simulink model "mppt"  (R2020a)
settings: Solver=ode15s  StartTime=0.0  StopTime=parameters.sim_duration  FixedStep=1e-8  MaxStep=1e-7  RelTol=1e-3
undefined symbols (not defined in the file or in its folder): Ion, Lithium, parameters, sigbuilder_block
libraries: powerlib x24, simulink x5, powerlib_meascontrol x2, electricdrivelib x1, dspswit3 x1, re_lib x1
settings Model: SimulationMode=accelerator  Creator=HP  LastModifiedBy=HP

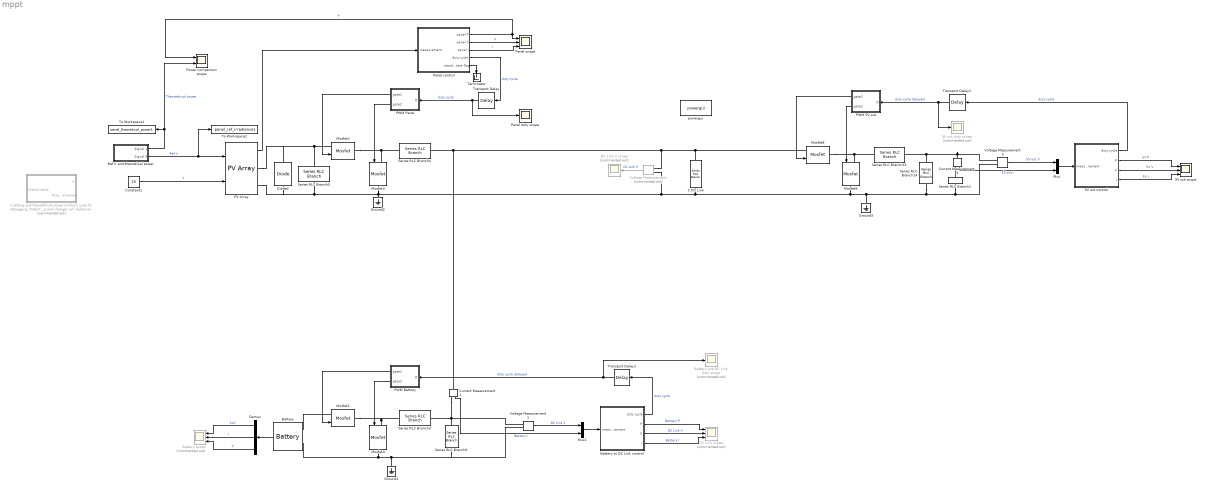
== system mppt ==
  5V out control : Subsystem
  5V out duty scope : Scope  Commented=on
  5V out scope : Scope  NumInputPorts=3
  Baterry scope : Scope  Commented=on  NumInputPorts=3
  Battery : electricdrivelib/Extra Sources/Battery  BatType=Lithium-Ion  ShowTempParam=off  ThermalPreset=no  ShowAgeParam=off  NomV=8  NomQ=2.6  SOC=50  Batt_Tr=30  PresetModel=off  MaxQ=2.6  MinV=6  FullV=9  Dis_rate=2.1304  R=0.019231  Normal_OP=2.3513  expZone="[8.5   2.12774]"  current=[6.5 13 32.5]  Units=Time  Tci=20  NomT=20  T2=-30  MaxQ2=4.8  FullV2=7.1  Normal_OP2=5.655  expZone2="[6.58           1]"  Rca=0.6  ti=2000  Dp=0  Neq0=0  Tsim=1e6  Ta1=25  Qeol=5.4*0.9  Reol=0.013333*1.2  Char_age=[2.3478, 3]  Dis_age=[2.3478, 10]  N1=1500  N2=10500  N3=1000  N4=1400  Ta2=45  N5=950
  Battery and DC Link duty scope : Scope  Commented=on
  Battery to DC Link control : Subsystem
  C DC Link : powerlib/Elements/Series RLC Branch  LConnTagsString=__new0  RConnTagsString=__new0  BranchType=RC  Resistance=0.01  Inductance=1e-3  SetiL0=off  InitialCurrent=0  Capacitance=400e-6  Setx0=off  InitialVoltage=0  Measurements=None
  Constant1 : Constant  Value=25
  Current Measurement1 : powerlib/Measurements/Current Measurement  PhasorSimulation=off  OutputType=Complex  PSBequivalent=0
  Current Measurement3 : powerlib/Measurements/Current Measurement  PhasorSimulation=off  OutputType=Complex  PSBequivalent=0
  DC Link V scope : Scope  Commented=on
  DC Link scope : Scope  Commented=on  NumInputPorts=3
  Demux : Demux  Outputs=3
  Diode2 : powerlib/Power Electronics/Diode  Ron=0.3  Lon=0  Vf=0.6  IC=0  UseSnubber=0  Rs=500  Cs=250e-9  Measurements=off
  Ground1 : powerlib/Elements/Ground  LConnTagsString=a
  Ground2 : powerlib/Elements/Ground  LConnTagsString=a
  Ground3 : powerlib/Elements/Ground  LConnTagsString=a
  Ir setting and theorethical power (A block used for debugging. Detects steady state and changes ref iradiance) : Subsystem  Commented=on
  Mosfet{1,4,8..9} (4 alike) : powerlib/Power Electronics/Mosfet  Ron=0.008  Lon=0  Rd=0.01  Vfd=1  IC=0  Rs=inf  Cs=inf  Measurements=off
  Mosfet2 : powerlib/Power Electronics/Mosfet  Ron=0.0029  Lon=0  Rd=0.01  Vfd=1  IC=0  Rs=inf  Cs=inf  Measurements=off
  Mosfet3 : powerlib/Power Electronics/Mosfet  Ron=0.0029  Lon=0  Rd=0.01  Vfd=1  IC=0  Rs=inf  Cs=inf  Measurements=off
  Mux : Mux  Inputs=2
  Mux1 : Mux  Inputs=2
  PV Array : re_lib/Solar/PV Array  Npar=1  Nser=1  PlotType=array @ 25 deg.C & specified irradiances  S_vec=[1000 800 500 400]  Temp_C_vec=[ 25 ]  ModuleName=User-defined  PlotWhenSelected=off  Pm=29.92  Ncell=36  Voc=21.9  Isc=1.84  Vm=17.6  Im=1.70  beta_Voc_pc=-0.33  alpha_Isc_pc=0.05  beta_Voc=-0.07227  alpha_Isc=0.00092  IL=1.8452  I0=2.0527e-11  nI=0.94005  Rsh=353.0773  Rs=1.0051  RobustModel=off  RobustCellTemperature=25  BAL=on  Tc=1e-8  Tfilter=5e-5
  PWM 5V out : Subsystem
  PWM Battery : Subsystem
  PWM Panel : Subsystem
  Panel control : Subsystem
  Panel duty scope : Scope
  Panel scope : Scope  NumInputPorts=3
  Power comparison scope : Scope  NumInputPorts=2
  Ref Ir and theoretical power : Subsystem  Tag=STV Subsys  LoadFcn=sigbuilder_block('load');  StartFcn=sigbuilder_block('start');  StopFcn=sigbuilder_block('stop');  ClipboardFcn=sigbuilder_block('clipboard');  mask(Sigbuilder block){tuvar=[0:10]}
      mask help: Simulink:masks:SigbuilderBlock_MD
      mask init:
      | if ~strcmp(get_param(bdroot(gcbh),'SimulationStatus'),'stopped') tuvar = sigbuilder_block('maskInit'); end
      settings: CopyFcn=sigbuilder_block('copy');  DeleteFcn=sigbuilder_block('delete');  ModelCloseFcn=sigbuilder_block('modelClose');  PreSaveFcn=sigbuilder_block('preSave');  PauseFcn=sigbuilder_block('pause');  ContinueFcn=sigbuilder_block('continue');  NameChangeFcn=sigbuilder_block('namechange');  OpenFcn=sigbuilder_block('open',[5.4 30 1141.2 522.6 ]);  CloseFcn=sigbuilder_block('close');
      mask Display: plot(0, 0, 100, 100,[2, 2, 32, 32, 2], [68, 8, 8, 68, 68],[32, 2], [38, 38], [32, 19, 2],[53, 60, 44], [32, 17, 17, 2],[16, 16, 31, 31]);txt = getActiveGroup(gcbh);text(2, 100, txt,'verticalAlignment', 'top');
  Series RLC Branch1 : powerlib/Elements/Series RLC Branch  LConnTagsString=__new0  RConnTagsString=__new0  BranchType=R  Resistance=2  Inductance=0  SetiL0=off  InitialCurrent=0  Capacitance=0  Setx0=off  InitialVoltage=0  Measurements=None
  Series RLC Branch13 : powerlib/Elements/Series RLC Branch  LConnTagsString=__new0  RConnTagsString=__new0  BranchType=RL  Resistance=0.01  Inductance=4.7e-6  SetiL0=off  InitialCurrent=0  Capacitance=1e-6  Setx0=off  InitialVoltage=0  Measurements=None
  Series RLC Branch14 : powerlib/Elements/Series RLC Branch  LConnTagsString=__new0  RConnTagsString=__new0  BranchType=RC  Resistance=0.01  Inductance=1e-3  SetiL0=off  InitialCurrent=0  Capacitance=47e-6  Setx0=off  InitialVoltage=0  Measurements=None
  Series RLC Branch3 : powerlib/Elements/Series RLC Branch  LConnTagsString=__new0  RConnTagsString=__new0  BranchType=RL  Resistance=0.01  Inductance=4.7e-6  SetiL0=off  InitialCurrent=0  Capacitance=1e-6  Setx0=off  InitialVoltage=0  Measurements=None
  Series RLC Branch4 : powerlib/Elements/Series RLC Branch  LConnTagsString=__new0  RConnTagsString=__new0  BranchType=RL  Resistance=0.009  Inductance=11.3e-6  SetiL0=off  InitialCurrent=0  Capacitance=1e-6  Setx0=off  InitialVoltage=0  Measurements=None
  Series RLC Branch5 : powerlib/Elements/Series RLC Branch  LConnTagsString=__new0  RConnTagsString=__new0  BranchType=RC  Resistance=0.01  Inductance=1e-3  SetiL0=off  InitialCurrent=0  Capacitance=22e-6  Setx0=off  InitialVoltage=0  Measurements=None
  Series RLC Branch6 : powerlib/Elements/Series RLC Branch  LConnTagsString=__new0  RConnTagsString=__new0  BranchType=RC  Resistance=0.01  Inductance=1e-3  SetiL0=off  InitialCurrent=0  Capacitance=47e-6  Setx0=off  InitialVoltage=0  Measurements=None
  Terminator : Terminator
  To Workspace1 : ToWorkspace  VariableName=panel_theoretical_power1  SaveFormat=Timeseries  SampleTime=-1
  To Workspace2 : ToWorkspace  VariableName=panel_ref_irradiance1  SaveFormat=Timeseries  SampleTime=-1
  Transport Delay : TransportDelay  DelayTime=parameters.transport_delay
  Transport Delay1 : TransportDelay  DelayTime=parameters.transport_delay
  Transport Delay2 : TransportDelay  DelayTime=parameters.transport_delay
  Voltage Measurement : powerlib/Measurements/Voltage Measurement  Commented=on  PhasorSimulation=off  OutputType=Complex  PSBequivalent=0
  Voltage Measurement1 : powerlib/Measurements/Voltage Measurement  PhasorSimulation=off  OutputType=Complex  PSBequivalent=0
  Voltage Measurement3 : powerlib/Measurements/Voltage Measurement  PhasorSimulation=off  OutputType=Complex  PSBequivalent=0
  powergui : powerlib/powergui  Priority=1  SimulationMode=Continuous  SampleTime=1e-8  frequency=60  Iterations=50  frequencyindice=0  Pbase=100e6  ErrMax=1e-4  UnitsV=kV  UnitsW=MW  buscounter=0  FunctionMessages=off  echomessages=off  EnableUseOfTLC=off  CurrentSourceSwitches=off  DisableSnubberDevices=off  DisableRonSwitches=off  DisableVfSwitches=off  DisplayEquations=off  AutomaticDiscreteSolvers=off  SolverType=Tustin/Backward Euler (TBE)  Interpol=off  ExternalGateDelay=off  methode=off  Ts=100  x0status=blocks  SPID=on  SwTol=0  HookPort=off  NonlinearTolerance=1e-4  nMaxIteration=100  ContinueOnMaxIteration=off  RestoreLinks=warning  ResistiveCurrentMeasurement=off  Frange=[0:2:500]  Ylog=off  Xlog=on  ShowGrid=off  save=off  variable=ZData  structure=0  ZoomFFT=off  StartTime=0.0  cycles=1  DisplayStyle=1  fundamental=60  FreqAxis=off  MaxFrequency=1000  frequencyindicesteady=1  RmsSteady=1  display=off
  wires:
  Constant1/1 -> PV Array/2  "T"
  PWM Panel/1(gate1) -> Mosfet2/1
  PWM Panel/2("gate2 ") -> Mosfet3/1
  PWM 5V out/1(gate1) -> Mosfet8/1
  Transport Delay2/1 -> PWM 5V out/1(D), 5V out duty scope/1  "duty cycle delayed"
  PWM 5V out/2("gate2 ") -> Mosfet9/1
  Voltage Measurement/1 -> DC Link V scope/1  "DC Link V"
  Panel control/1(panel P) -> Power comparison scope/1, Panel scope/1  "P"
  Panel control/2(panel V) -> Panel scope/2  "V"
  Panel control/3(panel I) -> Panel scope/3  "I"
  Panel control/4(duty cycle) -> Transport Delay/1  "duty cycle"
  5V out control/1(duty cycle) -> Transport Delay2/1  "duty cycle"
  Voltage Measurement3/1 -> Mux/1  "5V out V"
  Current Measurement3/1 -> Mux/2  "5V out I"
  Mux/1 -> 5V out control/1(measurement)
  5V out control/2(P) -> 5V out scope/1  "5V P"
  5V out control/3(V) -> 5V out scope/2  "5V V"
  5V out control/4(I) -> 5V out scope/3  "5V I"
  Battery/1 -> Demux/1
  Demux/1 -> Baterry scope/1  "SoC"
  Demux/2 -> Baterry scope/2  "I"
  Demux/3 -> Baterry scope/3  "V"
  Battery to DC Link control/3(V) -> DC Link scope/2  "DC Link V"
  Battery to DC Link control/1(duty cycle) -> Transport Delay1/1  "duty cycle"
  Current Measurement1/1 -> Mux1/2  "Battery I"
  Voltage Measurement1/1 -> Mux1/1  "DC Link V"
  Mux1/1 -> Battery to DC Link control/1(measurement)
  Transport Delay1/1 -> PWM Battery/1(D), Battery and DC Link duty scope/1  "duty cycle delayed"
  PWM Battery/1(gate1) -> Mosfet1/1
  Battery to DC Link control/4(I) -> DC Link scope/3  "Battery I"
  Battery to DC Link control/2(P) -> DC Link scope/1  "Battery P"
  PWM Battery/2("gate2 ") -> Mosfet4/1
  Transport Delay/1 -> PWM Panel/1(D), Panel duty scope/1  "duty cycle"
  PV Array/1 -> Panel control/1(measurement)
  Ref Ir and theoretical power/1(Signal 1) -> To Workspace1/1, Power comparison scope/2  "Theorethical power"
  Panel control/5(steady state flag) -> Terminator/1
  Ref Ir and theoretical power/2(Signal 3) -> To Workspace2/1, PV Array/1  "Ref ir"
  connections:
  Mosfet2/LConn1 -- Diode2/RConn1 -- PV Array/RConn1 -- Series RLC Branch5/LConn1
  Mosfet2/RConn1 -- Series RLC Branch4/RConn1 -- Mosfet3/LConn1
  Voltage Measurement3/LConn2 -- Series RLC Branch1/RConn1 -- Series RLC Branch14/RConn1 -- Ground3/LConn1 -- Mosfet9/RConn1 -- Voltage Measurement/LConn2 -- Mosfet3/RConn1 -- Ground2/LConn1 -- Diode2/LConn1 -- PV Array/RConn2 -- Series RLC Branch5/RConn1 -- C DC Link/RConn1
  Mosfet8/RConn1 -- Series RLC Branch13/RConn1 -- Mosfet9/LConn1
  Voltage Measurement3/LConn1 -- Current Measurement3/LConn1 -- Series RLC Branch13/LConn1 -- Series RLC Branch14/LConn1
  Current Measurement3/RConn1 -- Series RLC Branch1/LConn1
  C DC Link/LConn1 -- Mosfet8/LConn1 -- Voltage Measurement/LConn1 -- Current Measurement1/LConn1 -- Series RLC Branch4/LConn1
  Mosfet4/LConn1 -- Series RLC Branch3/RConn1 -- Mosfet1/RConn1
  Mosfet1/LConn1 -- Battery/LConn1
  Mosfet4/RConn1 -- Voltage Measurement1/LConn2 -- Series RLC Branch6/RConn1 -- Ground1/LConn1 -- Battery/LConn2
  Voltage Measurement1/LConn1 -- Current Measurement1/RConn1 -- Series RLC Branch3/LConn1 -- Series RLC Branch6/LConn1

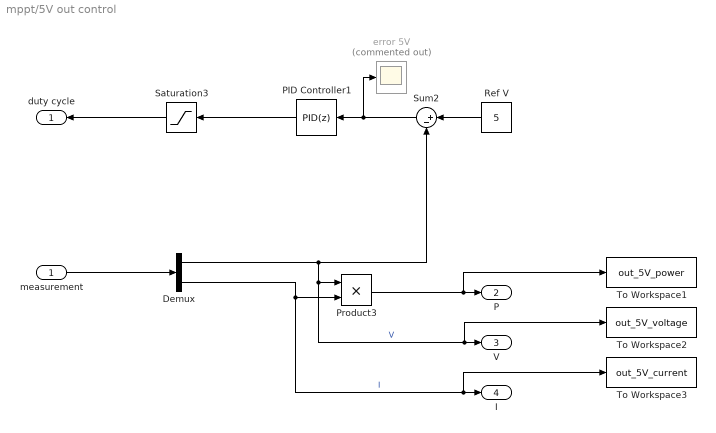
== system mppt/5V out control ==
  measurement : Inport
  Demux : Demux  Outputs=2
  PID Controller1 : simulink/Continuous/PID Controller  Controller=PID  Form=Parallel  TimeDomain=Discrete-time  UseExternalTs=off  SampleTime=parameters.sampling_time  IntegratorMethod=Forward Euler  FilterMethod=Forward Euler  ControllerParametersSource=internal  P=0.03  I=0.03*1e4  D=0  UseFilter=on  N=100  TunerSelectOption=Transfer Function Based (PID Tuner App)  InitialConditionSource=internal  InitialConditionForIntegrator=0  InitialConditionForFilter=0  DifferentiatorICPrevScaledInput=0  ExternalReset=none  TrackingMode=off  Kt=1  LimitOutput=off  UpperSaturationLimit=inf  LowerSaturationLimit=-inf  LinearizeAsGain=on  AntiWindupMode=none  Kb=1  POutMin=[]  POutMax=[]  IOutMin=[]  IOutMax=[]  DOutMin=[]  DOutMax=[]  NOutMin=[]  NOutMax=[]  SumOutMin=[]  SumOutMax=[]  SaturationOutMin=[]  SaturationOutMax=[]  PParamMin=[]  PParamMax=[]  IParamMin=[]  IParamMax=[]  DParamMin=[]  DParamMax=[]  NParamMin=[]  NParamMax=[]  KbParamMin=[]  KbParamMax=[]  KtParamMin=[]  KtParamMax=[]  KbOutMin=[]  KbOutMax=[]  KtOutMin=[]  KtOutMax=[]  IntegratorOutMin=[]  IntegratorOutMax=[]  FilterOutMin=[]  FilterOutMax=[]  SumI1OutMin=[]  SumI1OutMax=[]  SumI2OutMin=[]  SumI2OutMax=[]  SumI3OutMin=[]  SumI3OutMax=[]  SumI4OutMin=[]  SumI4OutMax=[]  SumDOutMin=[]  SumDOutMax=[]  DifferentiatorOutMin=[]  DifferentiatorOutMax=[]  FilterDiffOutCoefMin=[]  FilterDiffOutCoefMax=[]  ReciprocalOutMin=[]  ReciprocalOutMax=[]  SumDenOutMin=[]  SumDenOutMax=[]  SumNumOutMin=[]  SumNumOutMax=[]  DivideOutMin=[]  DivideOutMax=[]  UdiffTsProdOutMin=[]  UdiffTsProdOutMax=[]  NTsProdOutMin=[]  NTsProdOutMax=[]  UintegralTsProdOutMin=[]  UintegralTsProdOutMax=[]  UngainTsProdOutMin=[]  UngainTsProdOutMax=[]  IntegratorContinuousStateAttributes=''  IntegratorStateMustResolveToSignalObject=off  IntegratorRTWStateStorageClass=Auto  FilterContinuousStateAttributes=''  FilterStateMustResolveToSignalObject=off  FilterRTWStateStorageClass=Auto  ParallelPVariant=InternalParameters  IdealPVariant=Disabled  IVariant=InternalParameters  DVariant=InternalParameters  IntegratorVariant=Discrete  SatVariant=Disabled  AWVariant=Passthrough  PCopyVariant=Disabled  TRVariant=Disabled  FdbkBlocksVariant=Forward  IdealPFdbkVariant=Disabled  SatFdbkVariant=Disabled  DerivativeFilterVariant=ForwardEulerFilter  NVariant=InternalParameters  NCopyVariant=Disabled  FilterICVariant=InternalICsFilter  IntegratorICVariant=InternalICs  ExternalResetVariant=Disabled  TRSumVariant=Passthrough  SumFdbkVariant=Disabled  SumVariant=Sum_PID  TsampFilterVariant=InternalTs  TsampNgainVariant=Passthrough  TsampIntegralVariant=Passthrough
  Product3 : Product
  Ref V : Constant  Value=5
  Saturation3 : Saturate  UpperLimit=1  LowerLimit=0
  Sum2 : Sum  Inputs=|+-
  To Workspace1 : ToWorkspace  VariableName=out_5V_power  SaveFormat=Timeseries  SampleTime=-1
  To Workspace2 : ToWorkspace  VariableName=out_5V_voltage  SaveFormat=Timeseries  SampleTime=-1
  To Workspace3 : ToWorkspace  VariableName=out_5V_current  SaveFormat=Timeseries  SampleTime=-1
  error 5V : Scope  Commented=on
  duty cycle : Outport
  P : Outport  Port=2
  V : Outport  Port=3
  I : Outport  Port=4
  wires:
  Sum2/1 -> PID Controller1/1, error 5V/1
  PID Controller1/1 -> Saturation3/1
  Product3/1 -> To Workspace1/1, P/1
  Demux/1 -> Sum2/2, To Workspace2/1, V/1, Product3/1  "V"
  Ref V/1 -> Sum2/1
  Demux/2 -> To Workspace3/1, I/1, Product3/2  "I"
  Saturation3/1 -> duty cycle/1
  measurement/1 -> Demux/1

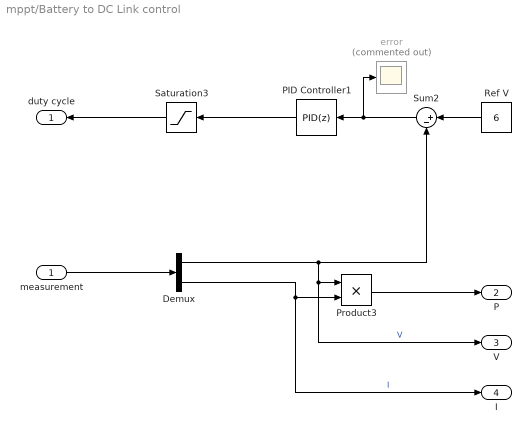
== system mppt/Battery to DC Link control ==
  measurement : Inport
  Demux : Demux  Outputs=2
  PID Controller1 : simulink/Continuous/PID Controller  Controller=PID  Form=Parallel  TimeDomain=Discrete-time  UseExternalTs=off  SampleTime=parameters.sampling_time  IntegratorMethod=Forward Euler  FilterMethod=Forward Euler  ControllerParametersSource=internal  P=0.03  I=0.03*1e4  D=0  UseFilter=on  N=100  TunerSelectOption=Transfer Function Based (PID Tuner App)  InitialConditionSource=internal  InitialConditionForIntegrator=0  InitialConditionForFilter=0  DifferentiatorICPrevScaledInput=0  ExternalReset=none  TrackingMode=off  Kt=1  LimitOutput=off  UpperSaturationLimit=inf  LowerSaturationLimit=-inf  LinearizeAsGain=on  AntiWindupMode=none  Kb=1  POutMin=[]  POutMax=[]  IOutMin=[]  IOutMax=[]  DOutMin=[]  DOutMax=[]  NOutMin=[]  NOutMax=[]  SumOutMin=[]  SumOutMax=[]  SaturationOutMin=[]  SaturationOutMax=[]  PParamMin=[]  PParamMax=[]  IParamMin=[]  IParamMax=[]  DParamMin=[]  DParamMax=[]  NParamMin=[]  NParamMax=[]  KbParamMin=[]  KbParamMax=[]  KtParamMin=[]  KtParamMax=[]  KbOutMin=[]  KbOutMax=[]  KtOutMin=[]  KtOutMax=[]  IntegratorOutMin=[]  IntegratorOutMax=[]  FilterOutMin=[]  FilterOutMax=[]  SumI1OutMin=[]  SumI1OutMax=[]  SumI2OutMin=[]  SumI2OutMax=[]  SumI3OutMin=[]  SumI3OutMax=[]  SumI4OutMin=[]  SumI4OutMax=[]  SumDOutMin=[]  SumDOutMax=[]  DifferentiatorOutMin=[]  DifferentiatorOutMax=[]  FilterDiffOutCoefMin=[]  FilterDiffOutCoefMax=[]  ReciprocalOutMin=[]  ReciprocalOutMax=[]  SumDenOutMin=[]  SumDenOutMax=[]  SumNumOutMin=[]  SumNumOutMax=[]  DivideOutMin=[]  DivideOutMax=[]  UdiffTsProdOutMin=[]  UdiffTsProdOutMax=[]  NTsProdOutMin=[]  NTsProdOutMax=[]  UintegralTsProdOutMin=[]  UintegralTsProdOutMax=[]  UngainTsProdOutMin=[]  UngainTsProdOutMax=[]  IntegratorContinuousStateAttributes=''  IntegratorStateMustResolveToSignalObject=off  IntegratorRTWStateStorageClass=Auto  FilterContinuousStateAttributes=''  FilterStateMustResolveToSignalObject=off  FilterRTWStateStorageClass=Auto  ParallelPVariant=InternalParameters  IdealPVariant=Disabled  IVariant=InternalParameters  DVariant=InternalParameters  IntegratorVariant=Discrete  SatVariant=Disabled  AWVariant=Passthrough  PCopyVariant=Disabled  TRVariant=Disabled  FdbkBlocksVariant=Forward  IdealPFdbkVariant=Disabled  SatFdbkVariant=Disabled  DerivativeFilterVariant=ForwardEulerFilter  NVariant=InternalParameters  NCopyVariant=Disabled  FilterICVariant=InternalICsFilter  IntegratorICVariant=InternalICs  ExternalResetVariant=Disabled  TRSumVariant=Passthrough  SumFdbkVariant=Disabled  SumVariant=Sum_PID  TsampFilterVariant=InternalTs  TsampNgainVariant=Passthrough  TsampIntegralVariant=Passthrough
  Product3 : Product
  Ref V : Constant  Value=6
  Saturation3 : Saturate  UpperLimit=1  LowerLimit=0
  Sum2 : Sum  Inputs=|+-
  "error " : Scope  Commented=on
  duty cycle : Outport
  P : Outport  Port=2
  V : Outport  Port=3
  I : Outport  Port=4
  wires:
  Sum2/1 -> PID Controller1/1, "error "/1
  PID Controller1/1 -> Saturation3/1
  Product3/1 -> P/1
  Demux/1 -> Sum2/2, V/1, Product3/1  "V"
  Ref V/1 -> Sum2/1
  Demux/2 -> I/1, Product3/2  "I"
  Saturation3/1 -> duty cycle/1
  measurement/1 -> Demux/1

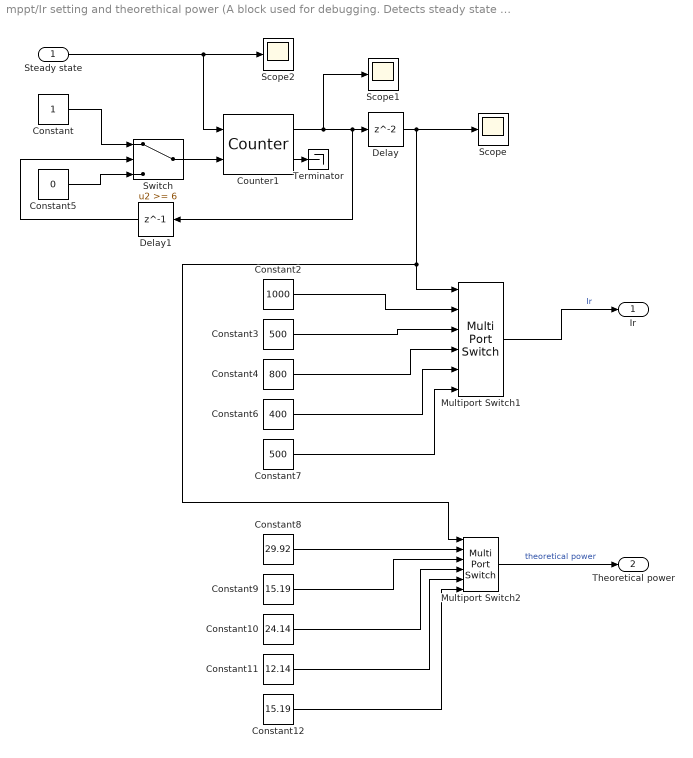
== system mppt/Ir setting and theorethical power (A block used for debugging. Detects steady state and changes ref iradiance) ==
  Steady state : Inport
  Constant : Constant
  Constant10 : Constant  Value=24.14
  Constant11 : Constant  Value=12.14
  Constant12 : Constant  Value=15.19
  Constant2 : Constant  Value=1000
  Constant3 : Constant  Value=500
  Constant4 : Constant  Value=800
  Constant5 : Constant  Value=0
  Constant6 : Constant  Value=400
  Constant7 : Constant  Value=500
  Constant8 : Constant  Value=29.92
  Constant9 : Constant  Value=15.19
  Counter1 : dspswit3/Counter  Direction=Up  CountEvent=Rising edge  CounterSize=User defined  MaxCount=255  InitialCount=1  Output=Count and Hit  HitValue=32  ResetInput=on  SamplesPerFrame=1  Ts=1  CntDtype=double  HitDtype=Logical
  Delay : Delay  InitialCondition=1
  Delay1 : Delay  DelayLength=1  InitialCondition=0
  Multiport Switch1 : MultiPortSwitch  Inputs=5
  Multiport Switch2 : MultiPortSwitch  Inputs=5
  Scope : Scope
  Scope1 : Scope
  Scope2 : Scope
  Switch : Switch  Threshold=6
  Terminator : Terminator
  Ir : Outport
  Theoretical power : Outport  Port=2
  wires:
  Constant9/1 -> Multiport Switch2/3
  Constant10/1 -> Multiport Switch2/4
  Delay/1 -> Multiport Switch1/1, Multiport Switch2/1, Scope/1
  Constant4/1 -> Multiport Switch1/4
  Constant11/1 -> Multiport Switch2/5
  Counter1/2 -> Terminator/1
  Constant/1 -> Switch/1
  Constant12/1 -> Multiport Switch2/6
  Counter1/1 -> Scope1/1, Delay1/1, Delay/1
  Constant8/1 -> Multiport Switch2/2
  Steady state/1 -> Scope2/1, Counter1/1
  Constant6/1 -> Multiport Switch1/5
  Constant5/1 -> Switch/3
  Constant7/1 -> Multiport Switch1/6
  Constant3/1 -> Multiport Switch1/3
  Constant2/1 -> Multiport Switch1/2
  Multiport Switch1/1 -> Ir/1  "Ir"
  Switch/1 -> Counter1/2
  Multiport Switch2/1 -> Theoretical power/1  "theoretical power"
  Delay1/1 -> Switch/2

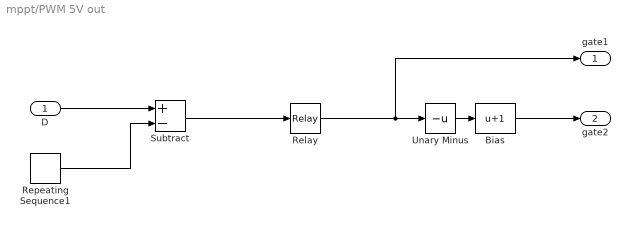
== system mppt/PWM 5V out ==
  D : Inport
  Bias : Bias  Bias=1
  Relay : Relay  OnSwitchValue=0  OffSwitchValue=0
  Repeating Sequence1 : simulink/Sources/Repeating Sequence  rep_seq_t=[0 1/300000]  rep_seq_y=[0 1]
  Subtract : Sum  Inputs=+-
  Unary Minus : UnaryMinus
  gate1 : Outport  VectorParamsAs1DForOutWhenUnconnected=off
  "gate2 " : Outport  Port=2  VectorParamsAs1DForOutWhenUnconnected=off
  wires:
  Relay/1 -> Unary Minus/1, gate1/1
  Subtract/1 -> Relay/1
  Unary Minus/1 -> Bias/1
  Bias/1 -> "gate2 "/1
  Repeating Sequence1/1 -> Subtract/2
  D/1 -> Subtract/1

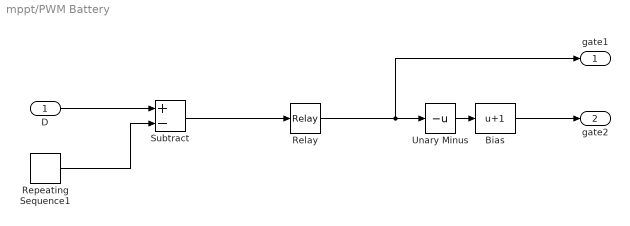
== system mppt/PWM Battery ==
  D : Inport
  Bias : Bias  Bias=1
  Relay : Relay  OnSwitchValue=0  OffSwitchValue=0
  Repeating Sequence1 : simulink/Sources/Repeating Sequence  rep_seq_t=[0 1/300000]  rep_seq_y=[0 1]
  Subtract : Sum  Inputs=+-
  Unary Minus : UnaryMinus
  gate1 : Outport  VectorParamsAs1DForOutWhenUnconnected=off
  "gate2 " : Outport  Port=2  VectorParamsAs1DForOutWhenUnconnected=off
  wires:
  Relay/1 -> Unary Minus/1, gate1/1
  Subtract/1 -> Relay/1
  Unary Minus/1 -> Bias/1
  Bias/1 -> "gate2 "/1
  Repeating Sequence1/1 -> Subtract/2
  D/1 -> Subtract/1

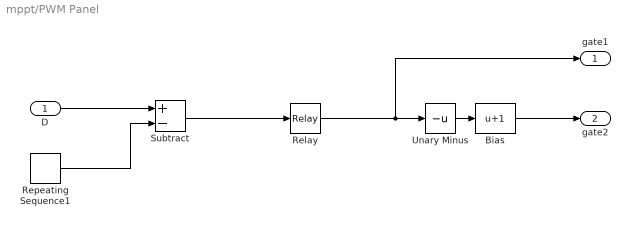
== system mppt/PWM Panel ==
  D : Inport
  Bias : Bias  Bias=1
  Relay : Relay  OnSwitchValue=0  OffSwitchValue=0
  Repeating Sequence1 : simulink/Sources/Repeating Sequence  rep_seq_t=[0 1/300000]  rep_seq_y=[0 1]
  Subtract : Sum  Inputs=+-
  Unary Minus : UnaryMinus
  gate1 : Outport  VectorParamsAs1DForOutWhenUnconnected=off
  "gate2 " : Outport  Port=2  VectorParamsAs1DForOutWhenUnconnected=off
  wires:
  Relay/1 -> Unary Minus/1, gate1/1
  Subtract/1 -> Relay/1
  Unary Minus/1 -> Bias/1
  Bias/1 -> "gate2 "/1
  Repeating Sequence1/1 -> Subtract/2
  D/1 -> Subtract/1

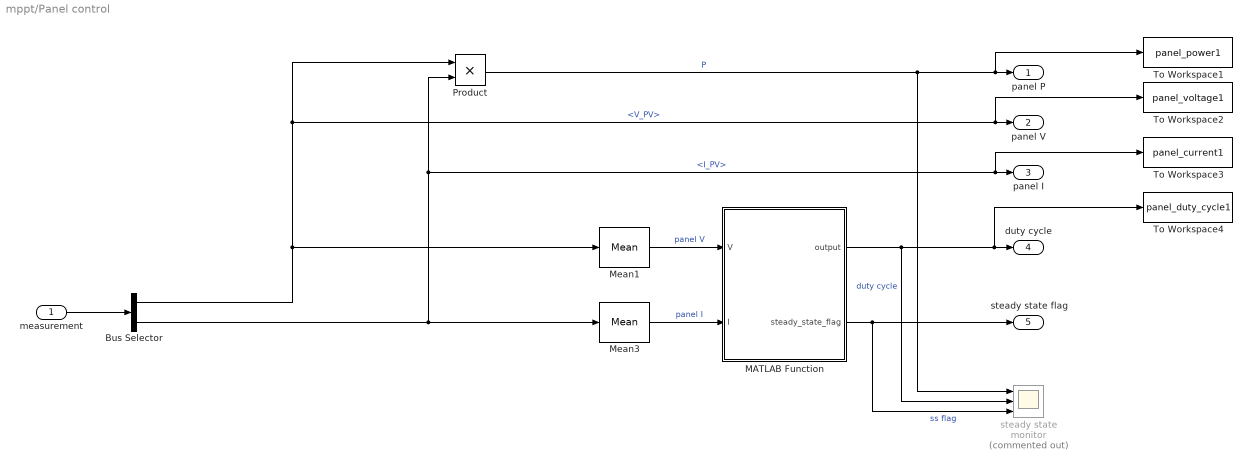
== system mppt/Panel control ==
  measurement : Inport
  Bus Selector : BusSelector  OutputSignals=V_PV,I_PV
  MATLAB Function : MATLAB Function  TreatAsAtomicUnit=on
  Mean1 : powerlib_meascontrol/Measurements/Mean  Freq=parameters.regulation_freq  Vinit=0  Ts=0
  Mean3 : powerlib_meascontrol/Measurements/Mean  Freq=parameters.regulation_freq  Vinit=0  Ts=0
  Product : Product
  To Workspace1 : ToWorkspace  VariableName=panel_power1  SaveFormat=Timeseries  SampleTime=-1
  To Workspace2 : ToWorkspace  VariableName=panel_voltage1  SaveFormat=Timeseries  SampleTime=-1
  To Workspace3 : ToWorkspace  VariableName=panel_current1  SaveFormat=Timeseries  SampleTime=-1
  To Workspace4 : ToWorkspace  VariableName=panel_duty_cycle1  SaveFormat=Timeseries  SampleTime=-1
  steady state monitor : Scope  Commented=on  NumInputPorts=3
  panel P : Outport
  panel V : Outport  Port=2
  panel I : Outport  Port=3
  duty cycle : Outport  Port=4
  steady state flag : Outport  Port=5
  wires:
  Mean3/1 -> MATLAB Function/2(I)  "panel I"
  Bus Selector/2 -> Mean3/1, Product/2, To Workspace3/1, panel I/1  "<I_PV>"
  Mean1/1 -> MATLAB Function/1(V)  "panel V"
  Bus Selector/1 -> To Workspace2/1, panel V/1, Product/1, Mean1/1  "<V_PV>"
  measurement/1 -> Bus Selector/1
  Product/1 -> steady state monitor/1, To Workspace1/1, panel P/1  "P"
  MATLAB Function/1(output) -> steady state monitor/2, To Workspace4/1, duty cycle/1  "duty cycle"
  MATLAB Function/2(steady_state_flag) -> steady state monitor/3, steady state flag/1  "ss flag"

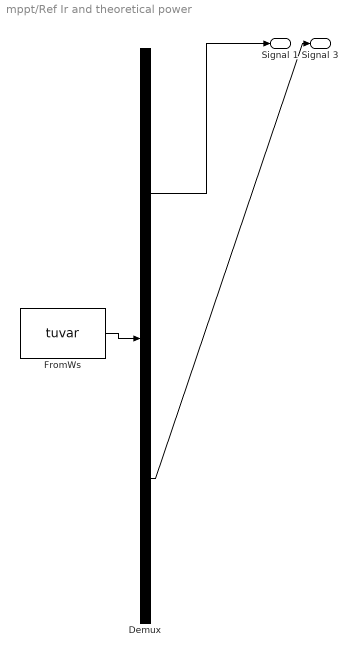
== system mppt/Ref Ir and theoretical power ==
  Demux : Demux  Tag=STV Demux  Outputs=2
      settings: DisplayOption=none
  FromWs : FromWorkspace  Tag=STV FromWs  VariableName=tuvar
      SigBuilderData=|
      | common.afterFinalStr = 'Extrapolate'
      | common.sampleTime = 0
      | dataSet.timeRange = [0 10]
      | dataSet.name = 'Group 1'
      | sbobj.Groups.Name = 'Group 1'
      | sbobj.Groups.Signals(1).Name = 'Signal 1'
      | sbobj.Groups.Signals(1).XData = [0 0.125 0.125 0.25 0.25 0.375 0.375 0.5 0.5 0.625 0.625 10]
      | sbobj.Groups.Signals(1).YData = [15.19 15.19 29.92 29.92 9.07 9.07 12.14 12.14 29.92 29.92 15.19 15.19]
      | sbobj.Groups.Signals(2).Name = 'Signal 3'
      | sbobj.Groups.Signals(2).XData = [0 0.125 0.125 0.25 0.25 0.375 0.375 0.5 0.5 0.625 0.625 10]
      | sbobj.Groups.Signals(2).YData = [500 500 1000 1000 300 300 400 400 1000 1000 500 500]
  Signal 1 : Outport  Tag=STV Outport
  Signal 3 : Outport  Tag=STV Outport  Port=2
  wires:
  FromWs/1 -> Demux/1
  Demux/1 -> Signal 1/1
  Demux/2 -> Signal 3/1

== matlab function mppt/Panel control/MATLAB Function ==
  settings: updateMethod=DISCRETE  sampleTime=parameters.sampling_time
  data: V input; output output; I input; parameters parameter; steady_state_flag output
function [output, steady_state_flag]  = mppt_algoritam(V, I, parameters)
    
    % parameters passed as 'parameter'
    % see editor->edit data->add and select parameter option!
    % useful stuff
    
    mppt_method = parameters.mppt_method;
    steady_state_flag = 0;
    output = 0;
    
    
    if mppt_method == 0
        [output, steady_state_flag] = QAlgoritam(V,I, parameters);
    else
        if mppt_method == 1
            output = ICAlgoritam(V, I);
        end
    end
    
end
